simulink model "Free_Flight"  (R2016a)
settings: configuration reference "AR_Drone_ConfigSet" (kept outside this file)
undefined symbols (not defined in the file or in its folder): accelerometerXyzGains, accelerometerXyzOffsets, DiscIntNeverNeededParam, Drone_StateModeType, fdesignblkfcn, gcbh, gyroXyzOffsets, Mag_Calib_Gain_Vector, Mag_Calib_Offset_Vector
libraries: simulink x7, AR_Drone_Sensors x3, AR_Drone_Actuators x2, vrlib x2, instrumentlib x1
(part 1 of 2)
settings Model: DataDictionary=ArDroneDataDictionary.sldd  SimulationMode=external  ExtModeTrigDuration=48000  Creator=nraman  LastModifiedBy=sbyebss
settings ConfigSetRef: DDName=ArDroneDataDictionary.sldd

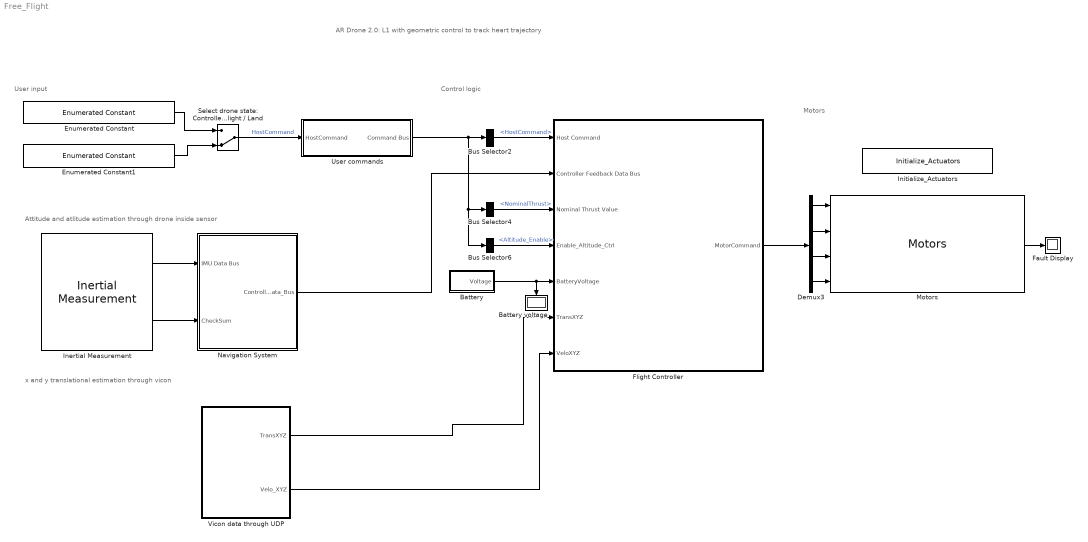
== system Free_Flight ==
  note: AR Drone 2.0: L1 with geometric control to track heart trajectory
  note: Motors
  note: Control logic
  note: x and y translational estimation through vicon
  note: User input
  note: Attitude and atlitude estimation through drone inside sensor
  Battery : Subsystem
  Battery voltage : Display
  Bus Selector2 : BusSelector  OutputSignals=HostCommand
  Bus Selector4 : BusSelector  OutputSignals=NominalThrust
  Bus Selector6 : BusSelector  OutputSignals=Altitude_Enable
  Demux3 : Demux
  Enumerated Constant : simulink/Sources/Enumerated Constant  OutDataTypeStr=Enum: Drone_StateModeType  Value=Drone_StateModeType.Controlled_Flight  SampleTime=inf
      settings: AttributesFormatString=%<Value>
  Enumerated Constant1 : simulink/Sources/Enumerated Constant  OutDataTypeStr=Enum: Drone_StateModeType  Value=Drone_StateModeType.Landing_Sequence  SampleTime=inf
      settings: AttributesFormatString=%<Value>
  Fault Display : Display
  Flight Controller : Subsystem  AncestorBlock=AR_Drone_Positioning/Flight Controller
  Inertial Measurement : AR_Drone_Sensors/Inertial Measurement  Ts=1/400
  Initialize_Actuators : AR_Drone_Actuators/Initialize_Actuators  ShowSpec=on
  Motors : AR_Drone_Actuators/Motors
  Navigation System : Subsystem  AncestorBlock=AR_Drone_Positioning/Navigation System
  Select drone state: Controlled Flight / Land : ManualSwitch  CurrentSetting=0
  User commands : Subsystem
  Vicon data through UDP : Subsystem
  wires:
  Motors/1 -> Fault Display/1
  Demux3/1 -> Motors/1
  Demux3/2 -> Motors/2
  Demux3/3 -> Motors/3
  Demux3/4 -> Motors/4
  Inertial Measurement/1 -> Navigation System/1(IMU Data Bus)
  Bus Selector4/1 -> Flight Controller/3(Nominal Thrust Value)  "<NominalThrust>"
  Bus Selector6/1 -> Flight Controller/4(Enable_Altitude_Ctrl)  "<Altitude_Enable>"
  Flight Controller/1(MotorCommand) -> Demux3/1
  Bus Selector2/1 -> Flight Controller/1(Host Command)  "<HostCommand>"
  Enumerated Constant/1 -> Select drone state: Controlled Flight / Land/1
  Enumerated Constant1/1 -> Select drone state: Controlled Flight / Land/2
  Battery/1(Voltage) -> Battery voltage/1, Flight Controller/5(BatteryVoltage)
  Inertial Measurement/2 -> Navigation System/2(CheckSum)
  User commands/1(Command Bus) -> Bus Selector6/1, Bus Selector4/1, Bus Selector2/1
  Select drone state: Controlled Flight / Land/1 -> User commands/1(HostCommand)  "HostCommand"
  Navigation System/1(Controller_Data_Bus) -> Flight Controller/2(Controller Feedback Data Bus)
  Vicon data through UDP/1("TransXYZ ") -> Flight Controller/6(TransXYZ)
  Vicon data through UDP/2(Velo_XYZ) -> Flight Controller/7(VeloXYZ)

== system Free_Flight/Battery ==
  Battery Voltage Measurement : AR_Drone_Sensors/Battery Voltage Measurement  SFunctionSpec=void BatteryMeasure_step(single y1[1])  SampleTime=-1
  Deci-Volts to Volts : Gain  Gain=1/10
  Voltage : Outport
  wires:
  Deci-Volts to Volts/1 -> Voltage/1
  Battery Voltage Measurement/1 -> Deci-Volts to Volts/1

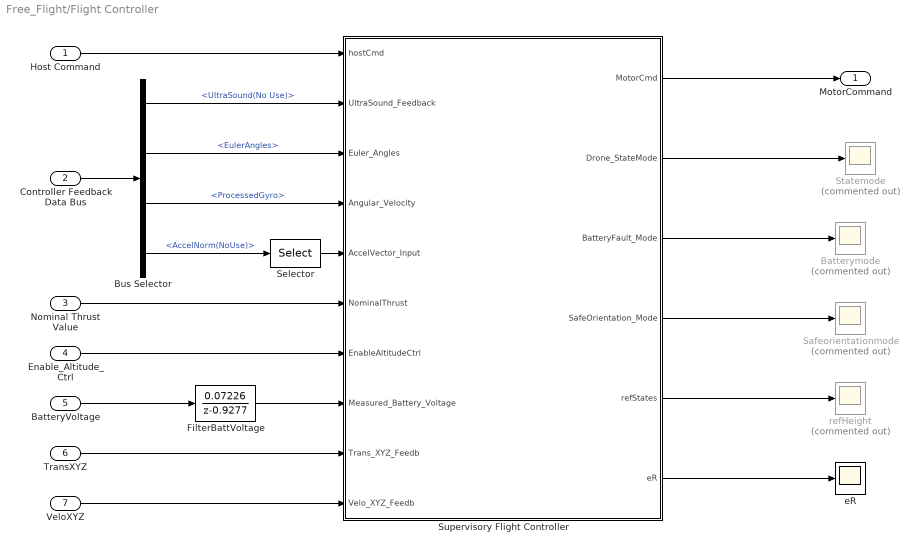
== system Free_Flight/Flight Controller ==
  Host Command : Inport
  Controller Feedback Data Bus : Inport  Port=2
  Nominal Thrust Value : Inport  Port=3
  Enable_Altitude_Ctrl : Inport  Port=4
  BatteryVoltage : Inport  Port=5
  TransXYZ : Inport  Port=6
  VeloXYZ : Inport  Port=7
  Batterymode : Scope  Commented=on
  Bus Selector : BusSelector  OutputSignals=UltraSound(No Use),EulerAngles,ProcessedGyro,AccelNorm(NoUse)
  FilterBattVoltage : DiscreteTransferFcn  Numerator=[ 0.07226]  Denominator=[1 -0.9277]
  Safeorientationmode : Scope  Commented=on
  Selector : Selector  InputPortWidth=3  IndexOptions=Index vector (dialog)  Indices=[3]  OutputSizes=1
  Statemode : Scope  Commented=on
  Supervisory Flight Controller : Stateflow chart  TreatAsAtomicUnit=on
  eR : Scope
  refHeight : Scope  Commented=on
  MotorCommand : Outport
  wires:
  Supervisory Flight Controller/5(refStates) -> refHeight/1
  Supervisory Flight Controller/4(" SafeOrientation_Mode") -> Safeorientationmode/1
  Supervisory Flight Controller/3(" BatteryFault_Mode") -> Batterymode/1
  Bus Selector/3 -> Supervisory Flight Controller/4(Angular_Velocity)  "<ProcessedGyro>"
  Bus Selector/2 -> Supervisory Flight Controller/3(Euler_Angles)  "<EulerAngles>"
  Bus Selector/4 -> Selector/1  "<AccelNorm(NoUse)>"
  Selector/1 -> Supervisory Flight Controller/5(AccelVector_Input)
  FilterBattVoltage/1 -> Supervisory Flight Controller/8(Measured_Battery_Voltage)
  BatteryVoltage/1 -> FilterBattVoltage/1
  Enable_Altitude_Ctrl/1 -> Supervisory Flight Controller/7(EnableAltitudeCtrl)
  Controller Feedback Data Bus/1 -> Bus Selector/1
  Nominal Thrust Value/1 -> Supervisory Flight Controller/6(NominalThrust)
  Bus Selector/1 -> Supervisory Flight Controller/2(UltraSound_Feedback)  "<UltraSound(No Use)>"
  Host Command/1 -> Supervisory Flight Controller/1(hostCmd)
  Supervisory Flight Controller/2(" Drone_StateMode") -> Statemode/1
  Supervisory Flight Controller/1(MotorCmd) -> MotorCommand/1
  TransXYZ/1 -> Supervisory Flight Controller/9(Trans_XYZ_Feedb)
  VeloXYZ/1 -> Supervisory Flight Controller/10(Velo_XYZ_Feedb)
  Supervisory Flight Controller/6(eR) -> eR/1

== system Free_Flight/Navigation System ==
  IMU Data Bus : Inport  OutDataTypeStr=Bus: IMU_Packets
  CheckSum : Inport  Port=2
  Bus Creator : BusCreator  Inputs=4
  Create Measurement Bus : Subsystem
  EulerAng : Scope
  Kalman Filter : Subsystem
  Measurement calibration correction : Subsystem
  Verify IMU Data : AR_Drone_Sensors/Verify IMU Data
  Controller_Data_Bus : Outport
  wires:
  Create Measurement Bus/1(Measurement Bus) -> Measurement calibration correction/1(MeasurementDataBus)
  Verify IMU Data/1 -> Create Measurement Bus/1(IMU Bus)
  Kalman Filter/3(AccelNorm_Ctrl) -> Bus Creator/4  "AccelNorm(NoUse)"
  Measurement calibration correction/1(Measurement_Calculation_Bus) -> Kalman Filter/1(Data_Bus)
  Bus Creator/1 -> Controller_Data_Bus/1
  Kalman Filter/1(UltraSound) -> Bus Creator/1  "UltraSound(No Use)"
  Kalman Filter/2(GyroDeg_Ctrl) -> Bus Creator/3  "ProcessedGyro"
  CheckSum/1 -> Verify IMU Data/2
  Kalman Filter/4(EulerAng_Ctrl) -> EulerAng/1, Bus Creator/2  "EulerAngles"
  IMU Data Bus/1 -> Verify IMU Data/1

== system Free_Flight/User commands ==
  HostCommand : Inport
  Altitude_OFF : Constant  Value=0
  Altitude_ON : Constant
  Bus Creator : BusCreator  Inputs=3
  Enable/Disable Altitude : ManualSwitch
  Nominal Thrust1 : Constant  Value=0
  Command Bus : Outport
  wires:
  Altitude_ON/1 -> Enable/Disable Altitude/1
  Altitude_OFF/1 -> Enable/Disable Altitude/2
  Nominal Thrust1/1 -> Bus Creator/2  "NominalThrust"
  HostCommand/1 -> Bus Creator/1  "HostCommand"
  Enable/Disable Altitude/1 -> Bus Creator/3  "Altitude_Enable"
  Bus Creator/1 -> Command Bus/1

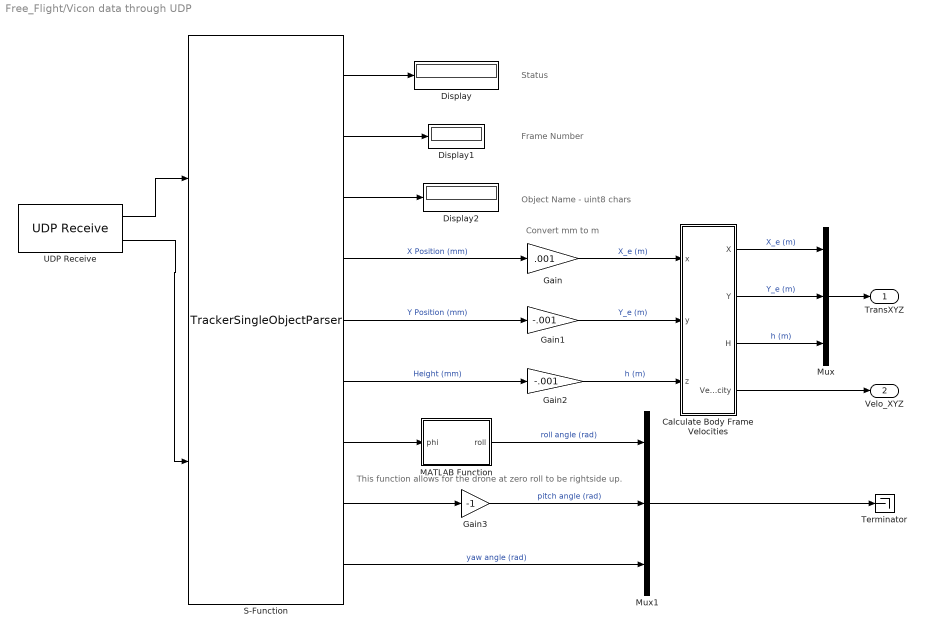
== system Free_Flight/Vicon data through UDP ==
  note: Object Name - uint8 chars
  note: Frame Number
  note: Status
  note: Convert mm to m
  note: This function allows for the drone at zero roll to be rightside up.
  Calculate Body Frame Velocities : Subsystem
  Display : Display
  Display1 : Display
  Display2 : Display
  Gain : Gain  Gain=.001
  Gain1 : Gain  Gain=-.001
  Gain2 : Gain  Gain=-.001
  Gain3 : Gain  Gain=-1  OutMin=-2.5  OutMax=2.5
  MATLAB Function : MATLAB Function  TreatAsAtomicUnit=on
  Mux : Mux  Inputs=3
  Mux1 : Mux  Inputs=3
  S-Function : S-Function  FunctionName=TrackerSingleObjectParser  Parameters='Object1'  SFunctionModules=TrackerSingleObjectParser  SFunctionDeploymentMode=off  EnableBusSupport=off
      settings: AttributesFormatString=Data Parser
  Terminator : Terminator
  UDP Receive : instrumentlib/UDP Receive  Priority=3  Host=localhost  Port=51001  LocalPort=51001  DataSize=256  EnableBlockingMode=off  Timeout=inf  SampleTime=0.01  DataType=uint8  ByteOrder=BigEndian
  "TransXYZ " : Outport
  Velo_XYZ : Outport  Port=2
  wires:
  UDP Receive/1 -> S-Function/1
  UDP Receive/2 -> S-Function/2
  S-Function/2 -> Display1/1
  S-Function/1 -> Display/1
  S-Function/3 -> Display2/1
  S-Function/6 -> Gain2/1  "Height (mm)"
  S-Function/5 -> Gain1/1  "Y Position (mm)"
  S-Function/4 -> Gain/1  "X Position (mm)"
  Calculate Body Frame Velocities/3(H) -> Mux/3  "h (m)"
  Calculate Body Frame Velocities/2(Y) -> Mux/2  "Y_e (m)"
  Calculate Body Frame Velocities/1(X) -> Mux/1  "X_e (m)"
  S-Function/9 -> Mux1/3  "yaw angle (rad)"
  Gain/1 -> Calculate Body Frame Velocities/1(x)  "X_e (m)"
  Gain1/1 -> Calculate Body Frame Velocities/2(y)  "Y_e (m)"
  Gain2/1 -> Calculate Body Frame Velocities/3(z)  "h (m)"
  S-Function/7 -> MATLAB Function/1(phi)
  MATLAB Function/1(roll) -> Mux1/1  "roll angle (rad)"
  Gain3/1 -> Mux1/2  "pitch angle (rad)"
  S-Function/8 -> Gain3/1
  Mux/1 -> "TransXYZ "/1
  Mux1/1 -> Terminator/1
  Calculate Body Frame Velocities/4(Velocity) -> Velo_XYZ/1

== system Free_Flight/Flight Controller/Supervisory Flight Controller/Attitude_Control ==
  note: Omega
  note: Comments on controller logic:
      | -The ARMED state should go HI right before take-off
      | -The  ARMED state should go LO in well after we have landed
      | -The ARMED state resets PI integrator when HI
      | -The ARMED state enables PI integrator when LO
  note: R:from body to inertial frame
      | Omega:roll,pitch,yaw=XYZ
  EulerAngle_Feedback_Deg : Inport  OutDataTypeStr=double  PortDimensions=3
  RateGyro_Feedback_Deg : Inport  Port=2  OutDataTypeStr=double  PortDimensions=3
  b3d : Inport  Port=3  OutDataTypeStr=double  PortDimensions=3
  f : TriggerPort  TriggerType=function-call  VariantControl=Variant
      settings: CopyFcn=Stateflow.SLINSF.SimulinkMan.removeBlockPreDeleteFcn  PreDeleteFcn=Stateflow.SLINSF.SimulinkMan.unsafePredeleteFcn
  Data Type Conversion2 : DataTypeConversion
  Eul2RotM : MATLAB Function  TreatAsAtomicUnit=on
  Rate Control : Subsystem
  Moment_controls : Outport  OutDataTypeStr=int16  PortDimensions=3  InitialOutput=0
  eR : Outport  Port=2  OutDataTypeStr=int16  PortDimensions=3  InitialOutput=0
  wires:
  EulerAngle_Feedback_Deg/1 -> Eul2RotM/1(EulAngs)
  Data Type Conversion2/1 -> Moment_controls/1
  b3d/1 -> Rate Control/1(b3d)
  RateGyro_Feedback_Deg/1 -> Rate Control/3(Omega)
  Eul2RotM/1(R) -> Rate Control/2(R)
  Rate Control/1(M) -> Data Type Conversion2/1
  Rate Control/2(eR) -> eR/1

== system Free_Flight/Flight Controller/Supervisory Flight Controller/Drone_State.Controlled_Flight.Altitude_Climb_Step1.E2R ==
  f : TriggerPort  TriggerType=function-call  VariantControl=Variant
      settings: CopyFcn=Stateflow.SLINSF.SimulinkMan.removeBlockPreDeleteFcn  PreDeleteFcn=Stateflow.SLINSF.SimulinkMan.unsafePredeleteFcn
  Clock : Clock
  Ref_pva : MATLAB Function  TreatAsAtomicUnit=on
  RefStates : Outport  OutDataTypeStr=int16
  wires:
  Clock/1 -> Ref_pva/1(t)
  Ref_pva/1(Ref) -> RefStates/1

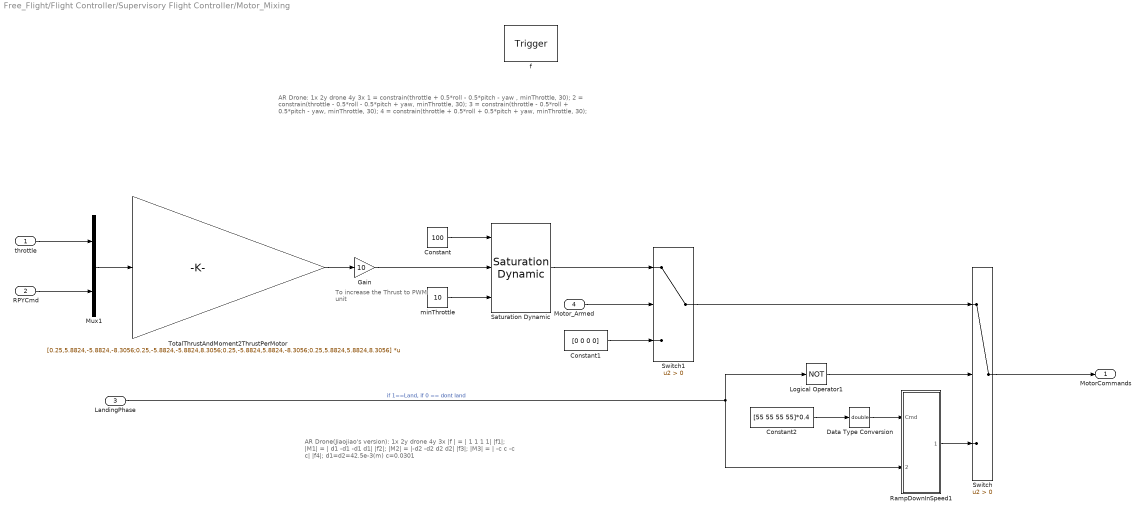
== system Free_Flight/Flight Controller/Supervisory Flight Controller/Motor_Mixing ==
  note: To increase the
      | Thrust to PWM unit
  note: AR Drone:
      |
      |   1x         2y
      |      drone
      |   4y         3x
      |
      |  1 = constrain(throttle + 0.5*roll - 0.5*pitch - yaw , minThrottle, 30);
      |  2 = constrain(throttle - 0.5*roll - 0.5*pitch + yaw, minThrottle, 30);
      |  3 = constrain(throttle - 0.5*roll + 0.5*pitch - yaw, minThrottle, 30);
      |  4 = constrain(throttle + 0.5*roll + 0.5*pitch + yaw, minThrottle, 30);
  note: AR Drone(Jiaojiao's version):
      |
      |   1x         2y
      |      drone
      |   4y         3x
      |
      |  |f | = |  1    1    1     1| |f1|;
      |  |M1| = | d1   -d1  -d1   d1| |f2|;
      |  |M2| = |-d2   -d2   d2   d2| |f3|;
      |  |M3| = | -c    c    -c    c| |f4|;
      |  d1=d2=42.5e-3(m)
      |  c=0.0301
  throttle : Inport  OutDataTypeStr=int16  PortDimensions=1
  RPYCmd : Inport  Port=2  OutDataTypeStr=int16  PortDimensions=3
  LandingPhase : Inport  Port=3  OutDataTypeStr=double  PortDimensions=1
  Motor_Armed : Inport  Port=4  OutDataTypeStr=double  PortDimensions=1
  f : TriggerPort  TriggerType=function-call  VariantControl=Variant
      settings: CopyFcn=Stateflow.SLINSF.SimulinkMan.removeBlockPreDeleteFcn  PreDeleteFcn=Stateflow.SLINSF.SimulinkMan.unsafePredeleteFcn
  Constant : Constant  Value=100  OutDataTypeStr=int16  SampleTime=-1
  Constant1 : Constant  Value=[0 0 0 0]  OutDataTypeStr=int16
  Constant2 : Constant  Value=[55 55 55 55]*0.4
  Data Type Conversion : DataTypeConversion  OutDataTypeStr=double
  Gain : Gain  Gain=10
  Logical Operator1 : Logic  Operator=NOT  AllPortsSameDT=off  OutDataTypeStr=boolean
  Mux1 : Mux  Inputs=2
  RampDownInSpeed1 : MATLAB Function  TreatAsAtomicUnit=on
  Saturation Dynamic : simulink/Discontinuities/Saturation Dynamic  OutMin=[]  OutMax=[]  OutDataTypeStr=Inherit: Same as second input  OutDataType=fixdt(1, 16)  OutScaling=2^-10  DoSatur=off
  Switch : Switch  Criteria=u2 > Threshold
  Switch1 : Switch  Criteria=u2 > Threshold
  TotalThrustAndMoment2ThrustPerMotor : Gain  Gain=[0.25,5.8824,-5.8824,-8.3056;0.25,-5.8824,-5.8824,8.3056;0.25,-5.8824,5.8824,-8.3056;0.25,5.8824,5.8824,8.3056]  Multiplication=Matrix(K*u)  ParamDataTypeStr=int16  OutDataTypeStr=int16
  minThrottle : Constant  Value=10  OutDataTypeStr=int16
  MotorCommands : Outport  InitialOutput=0
  wires:
  Switch1/1 -> Switch/1
  Constant1/1 -> Switch1/3
  Motor_Armed/1 -> Switch1/2
  Saturation Dynamic/1 -> Switch1/1
  Logical Operator1/1 -> Switch/2
  Switch/1 -> MotorCommands/1
  LandingPhase/1 -> Logical Operator1/1, RampDownInSpeed1/2(stopCmd)  "if 1==Land, if 0 == dont land"
  Constant2/1 -> Data Type Conversion/1
  RampDownInSpeed1/1(motorCmd) -> Switch/3
  Data Type Conversion/1 -> RampDownInSpeed1/1(Cmd)
  throttle/1 -> Mux1/1
  TotalThrustAndMoment2ThrustPerMotor/1 -> Gain/1
  Mux1/1 -> TotalThrustAndMoment2ThrustPerMotor/1
  Constant/1 -> Saturation Dynamic/1
  minThrottle/1 -> Saturation Dynamic/3
  RPYCmd/1 -> Mux1/2
  Gain/1 -> Saturation Dynamic/2

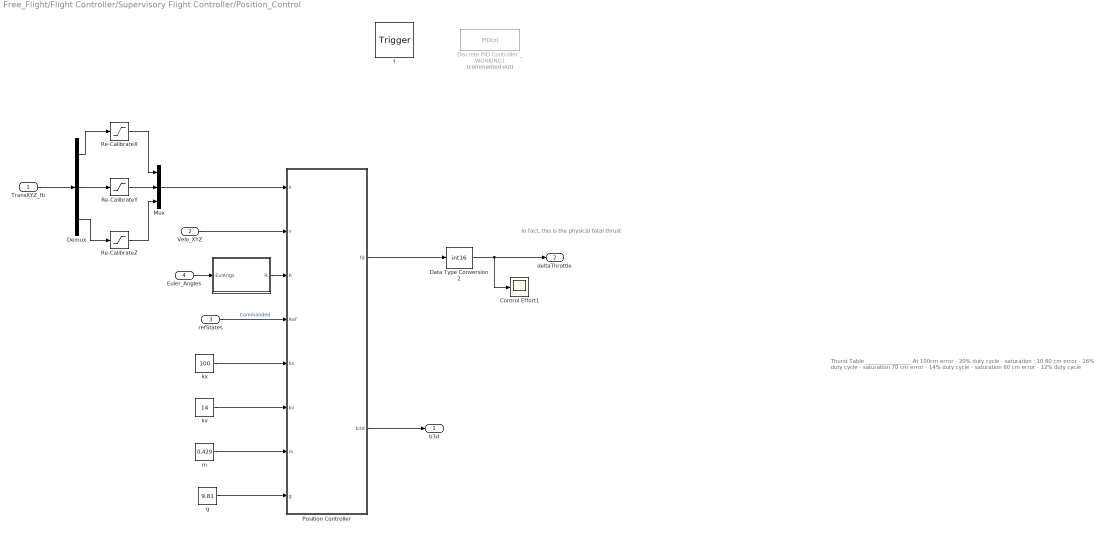
== system Free_Flight/Flight Controller/Supervisory Flight Controller/Position_Control ==
  note: In fact, this is the physical total thrust
  note: Thurst Table
      | _________________
      | At 100cm error  - 20% duty cycle - saturation : 10
      | 80 cm error - 16% duty cycle - saturation
      | 70 cm error - 14% duty cycle - saturation
      | 60 cm error - 12% duty cycle
  TransXYZ_fb : Inport  OutDataTypeStr=double  PortDimensions=3
  Velo_XYZ : Inport  Port=2  OutDataTypeStr=double  PortDimensions=1
  refStates : Inport  Port=3  OutDataTypeStr=double  PortDimensions=1
  Euler_Angles : Inport  Port=4  OutDataTypeStr=double  PortDimensions=3
  f : TriggerPort  TriggerType=function-call  VariantControl=Variant
      settings: CopyFcn=Stateflow.SLINSF.SimulinkMan.removeBlockPreDeleteFcn  PreDeleteFcn=Stateflow.SLINSF.SimulinkMan.unsafePredeleteFcn
  " " : MATLAB Function  TreatAsAtomicUnit=on
  Control Effort1 : Scope
  Data Type Conversion2 : DataTypeConversion  OutDataTypeStr=int16
  Demux : Demux  Outputs=3
  Discrete PID Controller _ WORKING1 : simulink/Continuous/PID Controller  Commented=on  Controller=PID  TimeDomain=Discrete-time  SampleTime=-1  IntegratorMethod=Forward Euler  FilterMethod=Forward Euler  Form=Parallel  UseFilter=on  ControllerParametersSource=internal  P=0.387369235850492*0.7  I=0.018136*4  D=0.819231727791919*0.15  N=12.5907330811849  InitialConditionSource=internal  InitialConditionForIntegrator=0  InitialConditionForFilter=0  ExternalReset=none  LimitOutput=on  UpperSaturationLimit=20  LowerSaturationLimit=-20  LinearizeAsGain=off  AntiWindupMode=clamping  Kb=1  TrackingMode=off  Kt=1  PParamMin=[]  PParamMax=[]  IParamMin=[]  IParamMax=[]  DParamMin=[]  DParamMax=[]  NParamMin=[]  NParamMax=[]  KbParamMin=[]  KbParamMax=[]  KtParamMin=[]  KtParamMax=[]  POutMin=[]  POutMax=[]  IOutMin=[]  IOutMax=[]  DOutMin=[]  DOutMax=[]  NOutMin=[]  NOutMax=[]  KbOutMin=[]  KbOutMax=[]  KtOutMin=[]  KtOutMax=[]  IntegratorOutMin=[]  IntegratorOutMax=[]  FilterOutMin=[]  FilterOutMax=[]  SumOutMin=[]  SumOutMax=[]  SumI1OutMin=[]  SumI1OutMax=[]  SumI2OutMin=[]  SumI2OutMax=[]  SumI3OutMin=[]  SumI3OutMax=[]  SumDOutMin=[]  SumDOutMax=[]  SaturationOutMin=[]  SaturationOutMax=[]  IntegratorContinuousStateAttributes=''  IntegratorStateMustResolveToSignalObject=off  IntegratorRTWStateStorageClass=Auto  FilterContinuousStateAttributes=''  FilterStateMustResolveToSignalObject=off  FilterRTWStateStorageClass=Auto  DifferentiatorICPrevScaledInput=0  DifferentiatorOutMin=[]  DifferentiatorOutMax=[]
  Mux : Mux  Inputs=3
  Position Controller : MATLAB Function  TreatAsAtomicUnit=on
  Re-CalibrateX : Saturate  UpperLimit=200  LowerLimit=0  OutMin=0  OutMax=200
      settings: AttributesFormatString=|
      | Upper: %<UpperLimit>
      | Lower %<LowerLimit>
  Re-CalibrateY : Saturate  UpperLimit=400  LowerLimit=-400  OutMin=-400  OutMax=400
      settings: AttributesFormatString=|
      | Upper: %<UpperLimit>
      | Lower %<LowerLimit>
  Re-CalibrateZ : Saturate  UpperLimit=400  LowerLimit=-400  OutMin=-400  OutMax=400
      settings: AttributesFormatString=|
      | Upper: %<UpperLimit>
      | Lower %<LowerLimit>
  g : Constant  Value=9.81
  kv : Constant  Value=14
  kx : Constant  Value=100
  m : Constant  Value=0.429
  b3d : Outport
  deltaThrottle : Outport  Port=2  OutDataTypeStr=int16
  wires:
  Re-CalibrateX/1 -> Mux/1
  Demux/1 -> Re-CalibrateX/1
  TransXYZ_fb/1 -> Demux/1
  Demux/2 -> Re-CalibrateY/1
  Demux/3 -> Re-CalibrateZ/1
  Re-CalibrateY/1 -> Mux/2
  Re-CalibrateZ/1 -> Mux/3
  Euler_Angles/1 -> " "/1(EulAngs)
  Mux/1 -> Position Controller/1(x)
  Velo_XYZ/1 -> Position Controller/2(v)
  refStates/1 -> Position Controller/4(Ref)  "Commanded"
  " "/1(R) -> Position Controller/3(R)
  kx/1 -> Position Controller/5(kx)
  kv/1 -> Position Controller/6(kv)
  m/1 -> Position Controller/7(m)
  g/1 -> Position Controller/8(g)
  Position Controller/2(b3d) -> b3d/1
  Position Controller/1(fd) -> Data Type Conversion2/1
  Data Type Conversion2/1 -> Control Effort1/1, deltaThrottle/1

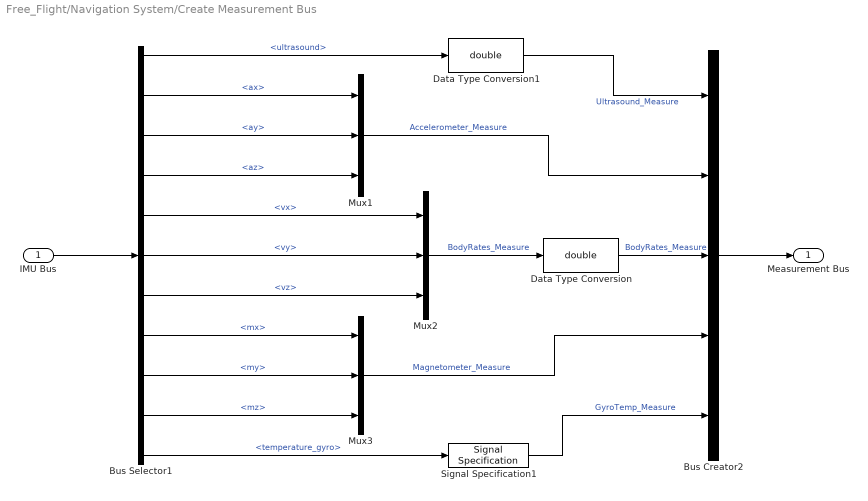
== system Free_Flight/Navigation System/Create Measurement Bus ==
  IMU Bus : Inport
  Bus Creator2 : BusCreator  Inputs=5
  Bus Selector1 : BusSelector  OutputSignals=ultrasound,ax,ay,az,vx,vy,vz,mx,my,mz,temperature_gyro
  Data Type Conversion : DataTypeConversion  OutDataTypeStr=double
  Data Type Conversion1 : DataTypeConversion  OutDataTypeStr=double
  Mux1 : Mux  Inputs=3
  Mux2 : Mux  Inputs=3
  Mux3 : Mux  Inputs=3
  Signal Specification1 : SignalSpecification
  Measurement Bus : Outport
  wires:
  Mux1/1 -> Bus Creator2/2  "Accelerometer_Measure"
  Bus Selector1/2 -> Mux1/1  "<ax>"
  Mux3/1 -> Bus Creator2/4  "Magnetometer_Measure"
  Data Type Conversion/1 -> Bus Creator2/3  "BodyRates_Measure"
  Bus Selector1/3 -> Mux1/2  "<ay>"
  Signal Specification1/1 -> Bus Creator2/5  "GyroTemp_Measure"
  Bus Selector1/4 -> Mux1/3  "<az>"
  Bus Selector1/9 -> Mux3/2  "<my>"
  Bus Selector1/10 -> Mux3/3  "<mz>"
  Bus Selector1/8 -> Mux3/1  "<mx>"
  IMU Bus/1 -> Bus Selector1/1
  Bus Selector1/5 -> Mux2/1  "<vx>"
  Bus Selector1/7 -> Mux2/3  "<vz>"
  Bus Selector1/6 -> Mux2/2  "<vy>"
  Bus Selector1/1 -> Data Type Conversion1/1  "<ultrasound>"
  Bus Selector1/11 -> Signal Specification1/1  "<temperature_gyro>"
  Data Type Conversion1/1 -> Bus Creator2/1  "Ultrasound_Measure"
  Bus Creator2/1 -> Measurement Bus/1
  Mux2/1 -> Data Type Conversion/1  "BodyRates_Measure"

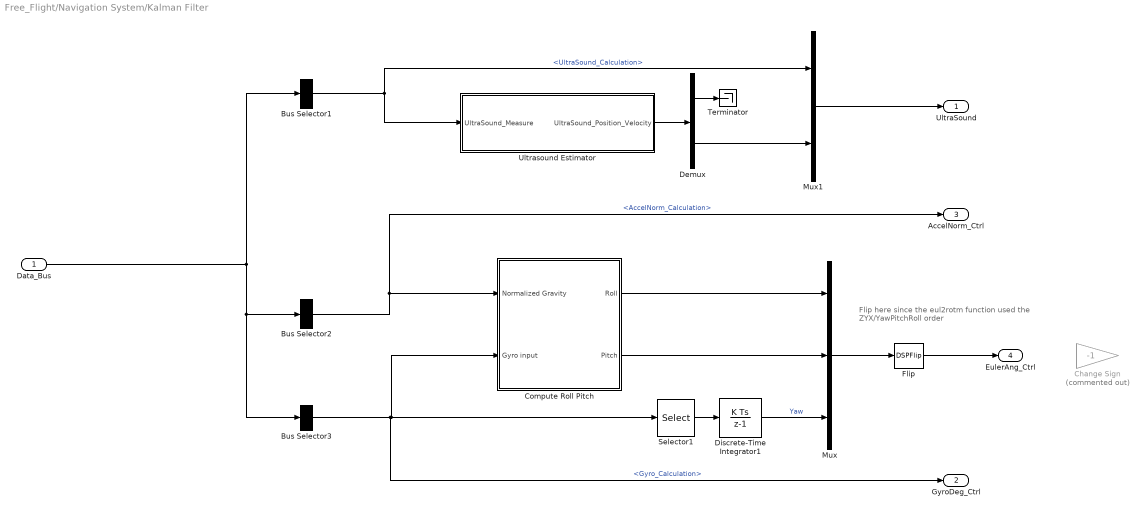
== system Free_Flight/Navigation System/Kalman Filter ==
  note: Flip here since the eul2rotm function
      | used the ZYX/YawPitchRoll order
  Data_Bus : Inport
  Bus Selector1 : BusSelector  OutputSignals=UltraSound_Calculation
  Bus Selector2 : BusSelector  OutputSignals=AccelNorm_Calculation
  Bus Selector3 : BusSelector  OutputSignals=Gyro_Calculation
  Change Sign : Gain  Commented=on  Gain=-1
  Compute Roll Pitch : Subsystem
  Demux : Demux  Outputs=2
  Discrete-Time Integrator1 : DiscreteIntegrator  SampleTime=-1  OutDataTypeStr=double  ICPrevOutput=DiscIntNeverNeededParam  ICPrevScaledInput=DiscIntNeverNeededParam
  Flip : DSPFlip
  Mux : Mux  Inputs=3
  Mux1 : Mux  Inputs=2
  Selector1 : Selector  IndexMode=Zero-based  InputPortWidth=3  IndexOptions=Index vector (dialog)  Indices=[2]  OutputSizes=1
  Terminator : Terminator
  Ultrasound Estimator : Subsystem
  UltraSound : Outport
  GyroDeg_Ctrl : Outport  Port=2
  AccelNorm_Ctrl : Outport  Port=3
  EulerAng_Ctrl : Outport  Port=4
  wires:
  Compute Roll Pitch/2(Pitch) -> Mux/2
  Compute Roll Pitch/1(Roll) -> Mux/1
  Selector1/1 -> Discrete-Time Integrator1/1
  Demux/1 -> Terminator/1
  Mux1/1 -> UltraSound/1
  Demux/2 -> Mux1/2
  Ultrasound Estimator/1("UltraSound_Position_Velocity ") -> Demux/1
  Bus Selector2/1 -> Compute Roll Pitch/1(Normalized Gravity), AccelNorm_Ctrl/1  "<AccelNorm_Calculation>"
  Discrete-Time Integrator1/1 -> Mux/3  "Yaw"
  Bus Selector3/1 -> GyroDeg_Ctrl/1, Selector1/1, Compute Roll Pitch/2(Gyro input)  "<Gyro_Calculation>"
  Data_Bus/1 -> Bus Selector1/1, Bus Selector2/1, Bus Selector3/1
  Bus Selector1/1 -> Ultrasound Estimator/1(UltraSound_Measure), Mux1/1  "<UltraSound_Calculation>"
  Mux/1 -> Flip/1
  Flip/1 -> EulerAng_Ctrl/1

== system Free_Flight/Navigation System/Measurement calibration correction ==
  MeasurementDataBus : Inport
  Accelerometer calibration : Subsystem
  Bus Creator1 : BusCreator  Inputs=4
  Bus Selector : BusSelector  OutputSignals=Ultrasound_Measure,Accelerometer_Measure,BodyRates_Measure,Magnetometer_Measure
  Calibration_Scale_and_Offset : Subsystem
  Gyro offset : Subsystem
  MATLAB Function : MATLAB Function  TreatAsAtomicUnit=on
  Measurement_Calculation_Bus : Outport
  wires:
  Bus Selector/1 -> MATLAB Function/1(Ultrasound_Measure)  "<Ultrasound_Measure>"
  Gyro offset/1(Gyro Offset Remove) -> Bus Creator1/3  "Gyro_Calculation"
  Bus Selector/2 -> Accelerometer calibration/1(Accel)  "<Accelerometer_Measure>"
  Accelerometer calibration/1(Accel_Norm) -> Bus Creator1/2  "AccelNorm_Calculation"
  MATLAB Function/1(UltraSound_Calculation) -> Bus Creator1/1  "UltraSound_Calculation"
  Calibration_Scale_and_Offset/1(Normalized  Magnetometer) -> Bus Creator1/4  "Magnetometer_Calculation"
  MeasurementDataBus/1 -> Bus Selector/1
  Bus Selector/3 -> Gyro offset/1(Raw Gyro Values)  "<BodyRates_Measure>"
  Bus Creator1/1 -> Measurement_Calculation_Bus/1
  Bus Selector/4 -> Calibration_Scale_and_Offset/1(RawMag)  "<Magnetometer_Measure>"

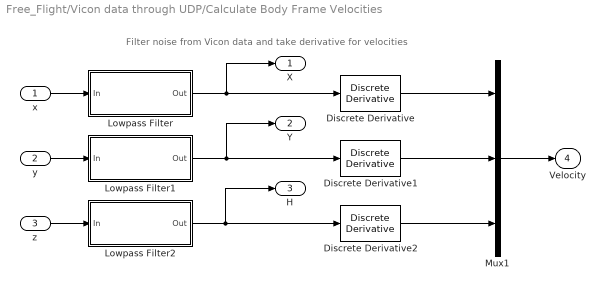
== system Free_Flight/Vicon data through UDP/Calculate Body Frame Velocities ==
  note: Filter noise from Vicon data and take derivative for velocities
  x : Inport
  y : Inport  Port=2
  z : Inport  Port=3
  Discrete Derivative : simulink/Discrete/Discrete Derivative  gainval=1.0  ICPrevScaledInput=0.0  InputProcessing=Inherited  OutMin=[]  OutMax=[]  OutDataType=fixdt(1, 16)  OutScaling=2^-10  DoSatur=off
  Discrete Derivative1 : simulink/Discrete/Discrete Derivative  gainval=1.0  ICPrevScaledInput=0.0  InputProcessing=Inherited  OutMin=[]  OutMax=[]  OutDataType=fixdt(1, 16)  OutScaling=2^-10  DoSatur=off
  Discrete Derivative2 : simulink/Discrete/Discrete Derivative  gainval=1.0  ICPrevScaledInput=0.0  InputProcessing=Inherited  OutMin=[]  OutMax=[]  OutDataType=fixdt(1, 16)  OutScaling=2^-10  DoSatur=off
  Lowpass Filter : Subsystem  DialogController=fdesignblkfcn  InitFcn=fdesignblkfcn(gcbh, {'InitFcn'});  mask(Lowpass Filter){}
      mask help: Design a lowpass filter
      settings: CopyFcn=fdesignblkfcn(gcbh, {'CopyFcn'});
      mask Help: helpview(mapfilelocation('dsp'), 'dsplowpassfilter');
      mask Display: disp('Lowpass')
  Lowpass Filter1 : Subsystem  DialogController=fdesignblkfcn  InitFcn=fdesignblkfcn(gcbh, {'InitFcn'});  mask(Lowpass Filter){}
      mask help: Design a lowpass filter
      settings: CopyFcn=fdesignblkfcn(gcbh, {'CopyFcn'});
      mask Help: helpview(mapfilelocation('dsp'), 'dsplowpassfilter');
      mask Display: disp('Lowpass')
  Lowpass Filter2 : Subsystem  DialogController=fdesignblkfcn  InitFcn=fdesignblkfcn(gcbh, {'InitFcn'});  mask(Lowpass Filter){}
      mask help: Design a lowpass filter
      settings: CopyFcn=fdesignblkfcn(gcbh, {'CopyFcn'});
      mask Help: helpview(mapfilelocation('dsp'), 'dsplowpassfilter');
      mask Display: disp('Lowpass')
  Mux1 : Mux  Inputs=3
  X : Outport
  Y : Outport  Port=2
  H : Outport  Port=3
  Velocity : Outport  Port=4
  wires:
  x/1 -> Lowpass Filter/1(In)
  Lowpass Filter/1(Out) -> X/1, Discrete Derivative/1
  y/1 -> Lowpass Filter1/1(In)
  Lowpass Filter1/1(Out) -> Y/1, Discrete Derivative1/1
  z/1 -> Lowpass Filter2/1(In)
  Lowpass Filter2/1(Out) -> H/1, Discrete Derivative2/1
  Mux1/1 -> Velocity/1
  Discrete Derivative2/1 -> Mux1/3
  Discrete Derivative1/1 -> Mux1/2
  Discrete Derivative/1 -> Mux1/1

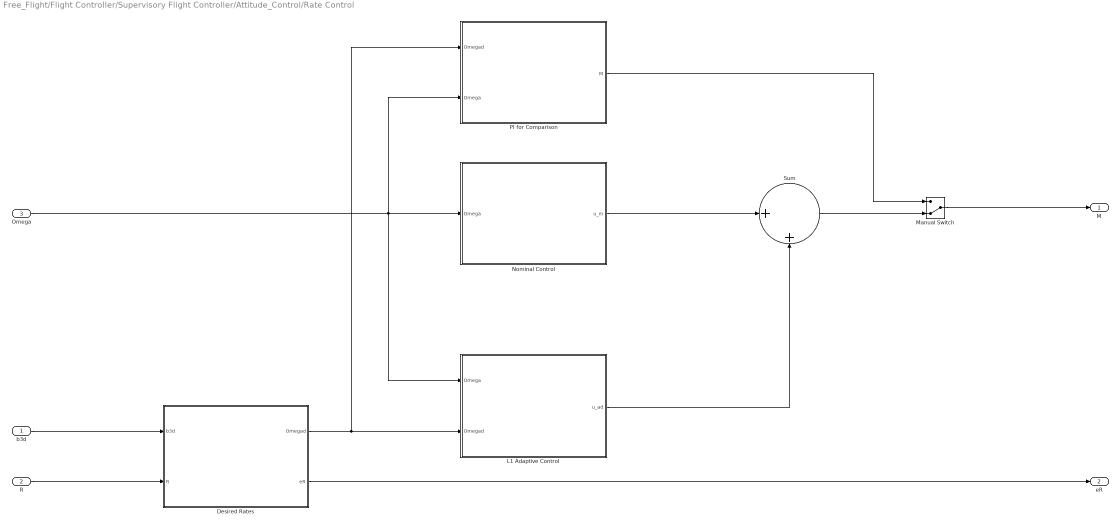
== system Free_Flight/Flight Controller/Supervisory Flight Controller/Attitude_Control/Rate Control ==
  b3d : Inport
  R : Inport  Port=2
  Omega : Inport  Port=3
  Desired Rates : Subsystem
  L1 Adaptive Control : Subsystem
  Manual Switch : ManualSwitch  CurrentSetting=0
  Nominal Control : Subsystem
  PI for Comparison : Subsystem
  Sum : Sum  Inputs=|++
  M : Outport
  eR : Outport  Port=2
  wires:
  b3d/1 -> Desired Rates/1(b3d)
  R/1 -> Desired Rates/2(R)
  Omega/1 -> PI for Comparison/2(Omega), L1 Adaptive Control/1(Omega), Nominal Control/1(Omega)
  Desired Rates/1(Omegad) -> PI for Comparison/1(Omegad), L1 Adaptive Control/2(Omegad)
  Desired Rates/2(eR) -> eR/1
  L1 Adaptive Control/1(u_ad) -> Sum/2
  Nominal Control/1(u_m) -> Sum/1
  Sum/1 -> Manual Switch/2
  Manual Switch/1 -> M/1
  PI for Comparison/1(M) -> Manual Switch/1

== system Free_Flight/Navigation System/Kalman Filter/Compute Roll Pitch ==
  Normalized Gravity : Inport
  Gyro input : Inport  Port=2
  Calculate Roll - Pitch : Subsystem
  KF_PITCH : Subsystem
  KF_ROLL : Subsystem
  Seperate Data : Subsystem
  Roll : Outport
  Pitch : Outport  Port=2
  wires:
  Seperate Data/1(Gyro_Roll_Ctrl) -> KF_ROLL/2(GYRO_ROLL_CTRL_IN)
  Seperate Data/2(Gyro_Pitch_Ctrl) -> KF_PITCH/1(GYRO_CTRL_IN)
  Calculate Roll - Pitch/1(RollRaw) -> KF_ROLL/1(ROLL_ACCEL_MEASURE)
  KF_ROLL/1(ROLL_FILTERED) -> Roll/1
  KF_PITCH/1(PITCH_FILTERED) -> Pitch/1  "Pitch"
  Calculate Roll - Pitch/2(PitchRaw) -> KF_PITCH/2(PITCH_ACCEL_MEASURE)
  Gyro input/1 -> Seperate Data/1(GyroIn)
  Normalized Gravity/1 -> Calculate Roll - Pitch/1(Normalized Gravity Vector)

== system Free_Flight/Navigation System/Kalman Filter/Ultrasound Estimator ==
  UltraSound_Measure : Inport
  Kalman Tracker : MATLAB Function  TreatAsAtomicUnit=on
  Unit Delay1 : UnitDelay  InitialCondition=[0 0 ]  SampleTime=-1
  Unit Delay2 : UnitDelay  InitialCondition=eye(2)  SampleTime=-1
  "UltraSound_Position_Velocity " : Outport
  wires:
  Unit Delay1/1 -> Kalman Tracker/3(state_correction_input), "UltraSound_Position_Velocity "/1
  Unit Delay2/1 -> Kalman Tracker/2(covariance_correction_input)
  UltraSound_Measure/1 -> Kalman Tracker/1(UltraSoundMeasure)
  Kalman Tracker/1(state_correction) -> Unit Delay1/1
  Kalman Tracker/2(covariance_correction) -> Unit Delay2/1

== system Free_Flight/Navigation System/Measurement calibration correction/Accelerometer calibration ==
  Accel : Inport
  Apply calibration parameters : Subsystem
  Data Type Conversion : DataTypeConversion  OutDataTypeStr=double
  Low pass filter : Subsystem
  Normalize Vector : vrlib/Utilities/Normalize Vector  maxzero=0
  Accel_Norm : Outport
  wires:
  Accel/1 -> Data Type Conversion/1
  Data Type Conversion/1 -> Apply calibration parameters/1(Raw Accelerometer Data)
  Apply calibration parameters/1(Calibrated Accelerometer Data) -> Low pass filter/1(Offset Accel)
  Low pass filter/1(Filtered Accel) -> Normalize Vector/1
  Normalize Vector/1 -> Accel_Norm/1

== system Free_Flight/Navigation System/Measurement calibration correction/Calibration_Scale_and_Offset ==
  RawMag : Inport
  Normalize Vector : vrlib/Utilities/Normalize Vector  maxzero=0
  Process Magnetometer : Subsystem
  Normalized  Magnetometer : Outport
  wires:
  RawMag/1 -> Process Magnetometer/1(Magnetometer)
  Process Magnetometer/1(MagVector) -> Normalize Vector/1
  Normalize Vector/1 -> Normalized  Magnetometer/1

== system Free_Flight/Navigation System/Measurement calibration correction/Gyro offset ==
  Raw Gyro Values : Inport
  Constant : Constant  Value=gyroXyzOffsets  VectorParams1D=off
  Demux : Demux  Outputs=3
  Demux1 : Demux  Outputs=3
  Mux1 : Mux  Inputs=3
  Process Raw Rate Gyro Data : Subsystem
  Sum : Sum  Inputs=|+-
  Sum1 : Sum  Inputs=|+-
  Sum2 : Sum  Inputs=|+-
  Gyro Offset Remove : Outport
  wires:
  Demux/3 -> Sum2/1
  Sum1/1 -> Mux1/2
  Demux1/1 -> Sum/2
  Sum2/1 -> Mux1/3
  Demux/2 -> Sum1/1
  Demux/1 -> Sum/1
  Sum/1 -> Mux1/1
  Mux1/1 -> Process Raw Rate Gyro Data/1(Raw Rate Gyro Data)
  Demux1/2 -> Sum1/2
  Demux1/3 -> Sum2/2
  Process Raw Rate Gyro Data/1(Processed Data) -> Gyro Offset Remove/1
  Constant/1 -> Demux1/1
  Raw Gyro Values/1 -> Demux/1

== system Free_Flight/Vicon data through UDP/Calculate Body Frame Velocities/Lowpass Filter ==
  In : Inport
  Generated Filter Block : DiscreteFir  Tag=BlockMethodSubSystem  Coefficients=[0.00055930462501575318 0.00013438735563549298 0.00015016454422028445 0.00016693857191824995 0.00018491342612616694 0.00020415963834189934 0.00022484753995734302 0.00024688855704748834 0.0002702509307130898 0.0002946787147561148 0.00032032059256713427 0.00034738161055017928 0.00037650323749600288 0.00040706323680379623 0.00043796983695636377 0.00047196663408886528 0.00050662961862923983 0.00054325840001079892 0.00058144666747780654 0.00062148347883108788 0.00066324011496819734 0.00070678679173187303 0.00075196662933983954 0.00079895723200710102 0.00084778697056723216 0.00089856743480663315 0.00095098680042624939 0.0010053609824103734 0.0010618954967739601 0.0011199925861139178 0.0011802526626944246 0.0012423196186075272 0.001306420024745494 0.0013724411094831683 0.0014404140081467152 0.0015102878259103543 0.0015821449091196669 0.0016559303131605751 0.0017316162508579831 0.0018091389420590142 0.0018886907963105563 0.0019700899150594323 0.0020532604439670635 0.0021383975552630632 0.0022252341005898385 0.0023139366140836953 0.0024043350087728744 0.0024964703414649399 0.0025902815032767088 0.0026857767291822315 0.0027828427108132943 0.0028814505503286479 0.0029815613431720561 0.0030831831249412203 0.0031861164566033065 0.0032904197190321924 0.0033960235082243001 0.0035027851957431444 0.0036107437056532663 0.0037197196047635242 0.0038297288508034786 0.0039406678666922112 0.0040524769811574055 0.0041650415992749157 0.0042783166767118731 0.0043922231969151558 0.0045066634941779288 0.004621505043287271 0.0047367581860537199 0.0048522536812996564 0.0049679238782070322 0.0050836955072573057 0.0051994152462688688 0.0053150586484085379 0.0054304744290612841 0.0055455813690235972 0.0056602646248898525 0.0057744530722521363 0.0058880260568144119 0.0060008663517301265 0.006112878298829021 0.0062239983039981527 0.0063340557168664637 0.0064430101899331316 0.0065507234705672046 0.006657097898589287 0.0067620598904020984 0.0068654617722319813 0.0069672290891802345 0.0070672553458439522 0.0071654534911182524 0.0072617072737138832 0.0073559174329184242 0.0074480105056045102 0.0075378834584868947 0.0076254188763999944 0.0077105717337323364 0.007793207924658074 0.007873278075044926 0.0079506864354509099 0.008025331653627581 0.0080971629689635116 0.0081660920354684457 0.0082320516118206087 0.0082949599720822213 0.0083547586175884876 0.0084113990338209547 0.0084647930001572128 0.0085148930300954582 0.0085616579958750251 0.0086050081057748775 0.0086449345827915702 0.0086813597923783657 0.0087142540447907972 0.0087435952038862307 0.0087693359025482667 0.0087914528339887998 0.0088099147152575219 0.0088247140503344146 0.0088358371788492714 0.0088432445604231091 0.0088469593598387887 0.0088469593598387887 0.0088432445604231091 0.0088358371788492714 0.0088247140503344146 0.0088099147152575219 0.0087914528339887998 0.0087693359025482667 0.0087435952038862307 0.0087142540447907972 0.0086813597923783657 0.0086449345827915702 0.0086050081057748775 0.0085616579958750251 0.0085148930300954582 0.0084647930001572128 0.0084113990338209547 0.0083547586175884876 0.0082949599720822213 0.0082320516118206087 0.0081660920354684457 0.0080971629689635116 0.008025331653627581 0.0079506864354509099 0.007873278075044926 0.007793207924658074 0.0077105717337323364 0.0076254188763999944 0.0075378834584868947 0.0074480105056045102 0.0073559174329184242 0.0072617072737138832 0.0071654534911182524 0.0070672553458439522 0.0069672290891802345 0.0068654617722319813 0.0067620598904020984 0.006657097898589287 0.0065507234705672046 0.0064430101899331316 0.0063340557168664637 0.0062239983039981527 0.006112878298829021 0.0060008663517301265 0.0058880260568144119 0.0057744530722521363 0.0056602646248898525 0.0055455813690235972 0.0054304744290612841 0.0053150586484085379 0.0051994152462688688 0.0050836955072573057 0.0049679238782070322 0.0048522536812996564 0.0047367581860537199 0.004621505043287271 0.0045066634941779288 0.0043922231969151558 0.0042783166767118731 0.0041650415992749157 ...(+1410 chars)]  InputProcessing=Columns as channels (frame based)
  Out : Outport
  wires:
  In/1 -> Generated Filter Block/1
  Generated Filter Block/1 -> Out/1

== system Free_Flight/Vicon data through UDP/Calculate Body Frame Velocities/Lowpass Filter1 ==
  In : Inport
  Generated Filter Block : DiscreteFir  Tag=BlockMethodSubSystem  Coefficients=[-0.00084475613175170818 1.9130153688269205e-05 2.0214131432315304e-05 2.1928029829354306e-05 2.4591858738332392e-05 2.7878622988662786e-05 3.2100156662285447e-05 3.6940303166599174e-05 4.2729969430913146e-05 4.9143314424989633e-05 5.6520563576693486e-05 6.4545533413592538e-05 7.3571517288272104e-05 8.3254688671381856e-05 9.3941922219367835e-05 0.00010534594669243068 0.00011780449047032596 0.00013096794104900143 0.00014525080846465319 0.00016028645933404204 0.00017646269948090235 0.00019342002126192381 0.00021160729603197307 0.00023058415946953592 0.00025084901215922608 0.00027191751714601312 0.00029437012506591527 0.00031761443557428771 0.00034235870055102373 0.00036783395721458236 0.00039502995575715097 0.00042255042896937006 0.0004518767762923991 0.00048418773030947649 0.00051494100809876275 0.00054804427989728853 0.00058213756218483681 0.00061784798315962655 0.00065471827305482928 0.00069306960413741407 0.00073268232761762358 0.00077372135005837758 0.00081609069746628189 0.00085987316503132968 0.00090503058209321838 0.00095156551328557011 0.00099951546818382751 0.001048892608257861 0.0010996728696636513 0.0011518531722417306 0.0012055015205849687 0.0012605253652633679 0.0013170110985270323 0.0013748814670609161 0.0014342292385452677 0.0014949162566170874 0.0015570882439231736 0.0016205791230290594 0.0016855629877502753 0.0017518110149012918 0.0018195615332199763 0.0018885122556354917 0.0019589932401155178 0.0020304857282480568 0.0021037769014525818 0.0021780809180233706 0.0022532033797941289 0.0023300764047560697 0.002408019136506376 0.0024872548308788127 0.0025675724927420509 0.0026490658254767325 0.0027316187670979935 0.0028152502306164374 0.0028999040138936419 0.0029855467479533273 0.0030721437562002806 0.0031596300441931848 0.0032480499708169006 0.0033372864419940786 0.0034272961291024195 0.0035180686103771725 0.0036095579990111323 0.0037016684075071105 0.0037944135684569395 0.0038876930607518608 0.0039814964276640866 0.004075711319748535 0.0041703660467547849 0.0042653206053666556 0.0043606048584123921 0.0044560567980269934 0.0045517449946426139 0.0046474690456441269 0.0047433220000064023 0.0048390514628438921 0.0049349409920054453 0.0050303599695821393 0.005125736595535545 0.0052209974723502455 0.0053158489890522886 0.0054103178039552891 0.0055043205657833117 0.0055978063251341924 0.005690716277565842 0.0057829693413471136 0.0058745343201712331 0.0059652981406936589 0.0060552512421996251 0.0061442804836209716 0.0062324255936591928 0.0063194439869470823 0.0064053997566050009 0.0064902080815222229 0.0065737893569911762 0.0066560643832651364 0.0067370215675464501 0.0068165448230662201 0.0068946139509815183 0.0069711333227454025 0.0070460960482252701 0.0071193815044052157 0.0071909886035725675 0.0072608058816287686 0.0073288500361475941 0.0073949837462685295 0.0074592372551665455 0.0075214871224524851 0.0075817908735233185 0.0076398465235371187 0.0076960193405338625 0.007749943492233664 0.0078016385772204976 0.0078510611899593914 0.0078982280680865644 0.007943044994299377 0.0079855298083864566 0.0080255928298220078 0.0080632614601325366 0.0080984370778125949 0.0081311701259260336 0.0081613666291623348 0.0081890712340489443 0.0082140625713304511 0.0082366057814709671 0.0082564961260276088 0.0082737716511510906 0.0082883995318900217 0.0083004112324183491 0.0083097353618941973 0.0083164213144566266 0.0083204210874554211 0.0083217726939814676 0.0083204210874554211 0.0083164213144566266 0.0083097353618941973 0.0083004112324183491 0.0082883995318900217 0.0082737716511510906 0.0082564961260276088 0.0082366057814709671 0.0082140625713304511 0.0081890712340489443 0.0081613666291623348 0.0081311701259260336 0.0080984370778125949 0.0080632614601325366 0.0080255928298220078 0.0079855298083864566 0.007943044994299377 0.0078982280680865644 0.0078510611899593914 0.0078016385772204976 0.007749943492233664 0.0076960193405338625 0.0076398465235371187 0.0075817908735233185 0.0075214871224524851 0.0074592372551665455 0.0073949837462685295 ...(+2792 chars)]  InputProcessing=Columns as channels (frame based)
  Out : Outport
  wires:
  In/1 -> Generated Filter Block/1
  Generated Filter Block/1 -> Out/1
